simulink model "mobile_robot_pathTracking"  (R2025b)
settings: Solver=ode1  StartTime=0.0  StopTime=120  FixedStep=0.1  RelTol=1e-3
model workspace (MAT data in the model file):
  example_omega_ts = timeseries
  example_omega_ts.Name = 'example_omega_ts'
  example_omega_ts.DataInfo = tsdata.datametadata
  example_omega_ts.DataInfo.Interpolation = tsdata.interpolation
  example_omega_ts.DataInfo.Interpolation.Fhandle : function handle (value not decoded)
  example_omega_ts.DataInfo.Interpolation.Name = 'linear'
  example_omega_ts.TimeInfo = tsdata.timemetadata
  example_omega_ts.TimeInfo.Length = 3001
  example_omega_ts.TimeInfo.DuplicateTimes = 0
  example_omega_ts.TimeInfo.Time_ = [0 0.02 0.04 0.06 0.08 0.1 0.12 0.14 0.16 0.18 0.2 0.22 ... (3001 elements, 3001x1)]
  example_omega_ts.TimeInfo.Initialized = 1
  example_omega_ts.QualityInfo = tsdata.qualmetadata
  example_omega_ts.Data_ = [0 0 0 0 0 0 0 0 0 0 0 0 ... (3001 elements, 3001x1)]
  example_v_ts = timeseries
  example_v_ts.Name = 'example_v_ts'
  example_v_ts.DataInfo = tsdata.datametadata
  example_v_ts.DataInfo.Interpolation = tsdata.interpolation
  example_v_ts.DataInfo.Interpolation.Fhandle : function handle (value not decoded)
  example_v_ts.DataInfo.Interpolation.Name = 'linear'
  example_v_ts.TimeInfo = tsdata.timemetadata
  example_v_ts.TimeInfo.Length = 3001
  example_v_ts.TimeInfo.DuplicateTimes = 0
  example_v_ts.TimeInfo.Time_ = [0 0.02 0.04 0.06 0.08 0.1 0.12 0.14 0.16 0.18 0.2 0.22 ... (3001 elements, 3001x1)]
  example_v_ts.TimeInfo.Initialized = 1
  example_v_ts.QualityInfo = tsdata.qualmetadata
  example_v_ts.Data_ = [0.25 0.25 0.25 0.25 0.25 0.25 0.25 0.25 0.25 0.25 0.25 0.25 ... (3001 elements, 3001x1)]
libraries: simulink x1
settings Model: PacingRate=10  Creator=Bender  LastModifiedBy=Bender

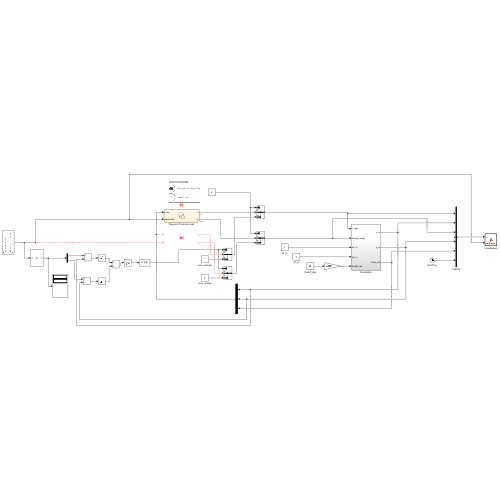
[thumbnail: Simulink's stored preview of the top-level diagram]
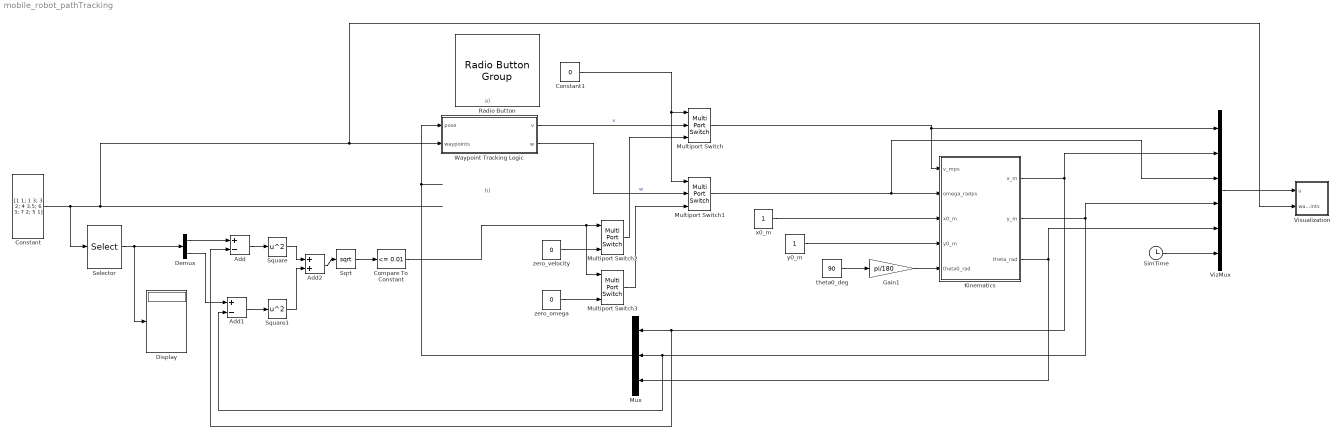
== system mobile_robot_pathTracking ==
  note: a)
  note: b)
  Add : Sum  Inputs=+-
  Add1 : Sum  Inputs=+-
  Add2 : Sum
  Compare To Constant : simulink/Logic and Bit Operations/Compare To Constant  relop=<=  const=0.01  OutDataTypeStr=boolean
  Constant : Constant  Value=[1 1; 1 3; 3 2; 4 3.5; 6 3; 7 2; 5 1]
  Constant1 : Constant  Value=0
  Demux : Demux  Outputs=2
  Display : Display
  Gain1 : Gain  Gain=pi/180
  Kinematics : Subsystem
  Multiport Switch{,1..3} (4 alike) : MultiPortSwitch  DataPortOrder=Zero-based contiguous  Inputs=2  zeroidx=on  SaturateOnIntegerOverflow=off  InputSameDT=off
  Mux : Mux  Inputs=3
  Radio Button : RadioButtonGroup  LabelPosition=Hide  SelectedLabel=P-Regler für Wegpunkte  ButtonGroupName=Bahnfolgeregelung
  Selector : Selector  NumberOfDimensions=2  InputPortWidth=2  IndexOptions=Index vector (dialog),Select all  Indices=[7],[7,2]  OutputSizes=1,1
  SimTime : Clock
  Sqrt : Sqrt
  Square : Math  Operator=square
  Square1 : Math  Operator=square
  Visualization : MATLAB Function  TreatAsAtomicUnit=on
  VizMux : Mux  Inputs=6
  Waypoint Tracking Logic : Stateflow chart  TreatAsAtomicUnit=on
  theta0_deg : Constant  Value=90
  x0_m : Constant
  y0_m : Constant
  zero_omega : Constant  Value=0
  zero_velocity : Constant  Value=0
  wires:
  SimTime/1 -> VizMux/6
  Kinematics/1(x_m) -> Add/2, Mux/1, VizMux/2
  Kinematics/2(y_m) -> Add1/2, Mux/2, VizMux/4
  Kinematics/3(theta_rad) -> Mux/3, VizMux/5
  VizMux/1 -> Visualization/1(u)
  x0_m/1 -> Kinematics/3(x0_m)
  y0_m/1 -> Kinematics/4(y0_m)
  theta0_deg/1 -> Gain1/1
  Gain1/1 -> Kinematics/5(theta0_rad)
  Mux/1 -> Waypoint Tracking Logic/1(pose)
  Multiport Switch2/1 -> Multiport Switch/3
  Multiport Switch3/1 -> Multiport Switch1/3
  Constant1/1 -> Multiport Switch/1, Multiport Switch1/1
  Waypoint Tracking Logic/1(v) -> Multiport Switch/2  "v"
  Waypoint Tracking Logic/2(w) -> Multiport Switch1/2  "w"
  Multiport Switch/1 -> VizMux/1, Kinematics/1(v_mps)
  Multiport Switch1/1 -> Kinematics/2(omega_radps), VizMux/3
  Constant/1 -> Selector/1, Visualization/2(waypoints), Waypoint Tracking Logic/2(waypoints)
  Selector/1 -> Demux/1, Display/1
  Demux/1 -> Add/1
  Demux/2 -> Add1/1
  Add/1 -> Square/1
  Square/1 -> Add2/1
  Add1/1 -> Square1/1
  Square1/1 -> Add2/2
  Add2/1 -> Sqrt/1
  Sqrt/1 -> Compare To Constant/1
  Compare To Constant/1 -> Multiport Switch3/1, Multiport Switch2/1
  ? -> Multiport Switch2/2
  zero_velocity/1 -> Multiport Switch2/3
  zero_omega/1 -> Multiport Switch3/3
  ? -> Multiport Switch3/2

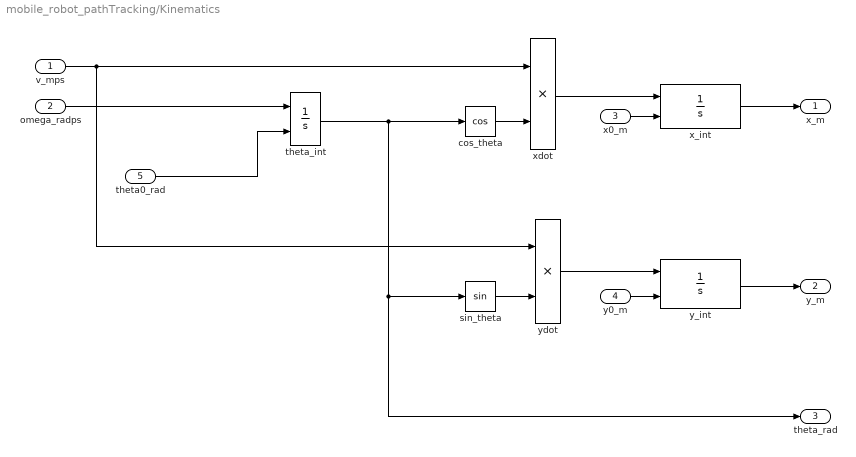
== system mobile_robot_pathTracking/Kinematics ==
  v_mps : Inport
  omega_radps : Inport  Port=2
  x0_m : Inport  Port=3
  y0_m : Inport  Port=4
  theta0_rad : Inport  Port=5
  cos_theta : Trigonometry  Operator=cos
  sin_theta : Trigonometry
  theta_int : Integrator  InitialConditionSource=external  InitialCondition=pi/2
  x_int : Integrator  InitialConditionSource=external  InitialCondition=1  LimitOutput=on  UpperSaturationLimit=8  LowerSaturationLimit=0
  xdot : Product
  y_int : Integrator  InitialConditionSource=external  InitialCondition=1  LimitOutput=on  UpperSaturationLimit=4  LowerSaturationLimit=0
  ydot : Product
  x_m : Outport
  y_m : Outport  Port=2
  theta_rad : Outport  Port=3
  wires:
  theta_int/1 -> sin_theta/1, theta_rad/1, cos_theta/1
  v_mps/1 -> xdot/1, ydot/1
  cos_theta/1 -> xdot/2
  sin_theta/1 -> ydot/2
  xdot/1 -> x_int/1
  ydot/1 -> y_int/1
  x_int/1 -> x_m/1
  y_int/1 -> y_m/1
  omega_radps/1 -> theta_int/1
  x0_m/1 -> x_int/2
  y0_m/1 -> y_int/2
  theta0_rad/1 -> theta_int/2

== matlab function mobile_robot_pathTracking/Visualization ==
  data: u input; waypoints input
function fcn(u, waypoints)
%#codegen
coder.extrinsic('robot_viz_update');
robot_viz_update(u, waypoints);
end

== stateflow chart mobile_robot_pathTracking/Waypoint Tracking Logic ==
  state FollowWaypoints
    entry:
    goalPoint = waypoints(idx,:);
    entry, during:
    [angle,range] = trackGoal(goalPoint);
    % TODO a): P-Regler
    w = 0;
  state ReachedGoal
    entry:
    v = 0;
    w = 0.3;
  (default) -> FollowWaypoints : {
      | v = 0.2;
      | idx = 1;
      | numPts = size(waypoints,1);
      | }
  FollowWaypoints -> (junction 39) : % Check if goal reached
      | [range < 0.1]
  (junction 39) -> ReachedGoal [order 1] : % Stop if final waypoint
      | [idx == numPts]
  (junction 39) -> (junction 42) [order 2]
  (junction 42) -> FollowWaypoints : % Go to the next waypoint
      | {idx = idx + 1;}
  data: goal function_input; ang function_output; dist function_output; pose input; waypoints input; v output; w output; angle local; range local; idx local; numPts local; goalPoint local
  function [ang,dist] = trackGoal(goal):
    | function [ang,dist] = trackGoal(goal)
    | % Finds the angle (theta) and distance (dist) between the 
    | % vehicle and a goal point
    |     
    | posDiff = [goal(1)-pose(1);goal(2)-pose(2)];
    | 
    | ang = angdiff(pose(3),atan2(posDiff(2),posDiff(1)));
    | dist = sqrt(posDiff(1)^2 + posDiff(2)^2);
